simulink model "bicycle"  (R2014b)
settings: Solver=ode45  StartTime=0.0  StopTime=50  RelTol=1e-3
settings Model: Creator=Prajwal  LastModifiedBy=Prajwal

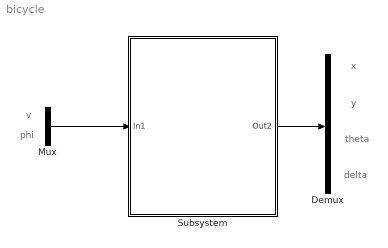
== system bicycle ==
  note: phi
  note: v
  note: delta
  note: theta
  note: y
  note: x
  Demux : Demux
  Mux : Mux  Inputs=2
  Subsystem : Subsystem
  wires:
  Subsystem/1(Out2) -> Demux/1
  Mux/1 -> Subsystem/1(In1)

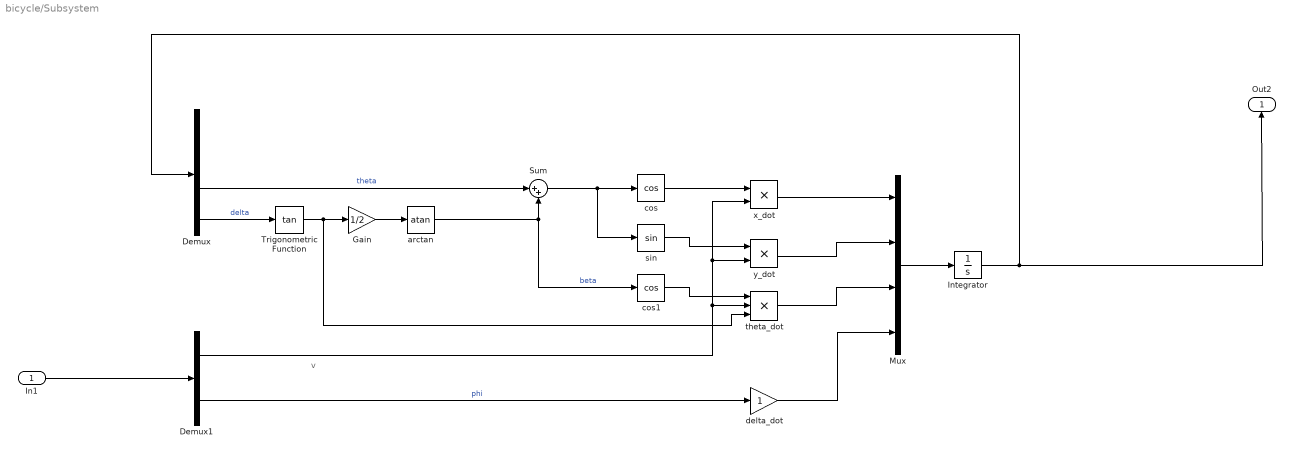
== system bicycle/Subsystem ==
  note: v
  In1 : Inport
  Demux : Demux
  Demux1 : Demux  Outputs=2
  Gain : Gain  Gain=1/2
  Integrator : Integrator  InitialCondition=[0 0 0 0]
  Mux : Mux
  Sum : Sum  Inputs=|++
  Trigonometric Function : Trigonometry  Operator=tan
  "arctan " : Trigonometry  Operator=atan
  cos : Trigonometry  Operator=cos
  cos1 : Trigonometry  Operator=cos
  delta_dot : Gain
  "sin " : Trigonometry
  theta_dot : Product  Inputs=3
  x_dot : Product
  y_dot : Product
  Out2 : Outport
  wires:
  theta_dot/1 -> Mux/3
  x_dot/1 -> Mux/1
  delta_dot/1 -> Mux/4
  Demux/4 -> Trigonometric Function/1  "delta"
  Demux/3 -> Sum/1  "theta"
  Integrator/1 -> Out2/1, Demux/1
  "arctan "/1 -> cos1/1, Sum/2  "beta"
  Demux1/2 -> delta_dot/1  "phi"
  In1/1 -> Demux1/1
  Mux/1 -> Integrator/1
  cos1/1 -> theta_dot/1
  y_dot/1 -> Mux/2
  Demux1/1 -> x_dot/2, y_dot/2, theta_dot/2
  Trigonometric Function/1 -> theta_dot/3, Gain/1
  Gain/1 -> "arctan "/1
  cos/1 -> x_dot/1
  Sum/1 -> cos/1, "sin "/1
  "sin "/1 -> y_dot/1
